simulink model "fuzzy_PD"  (R2022b)
settings: Solver=VariableStepAuto  StartTime=0.0  StopTime=400  RelTol=1e-3
libraries: fuzblock x1
settings Model: Creator=sophy  LastModifiedBy=sophy

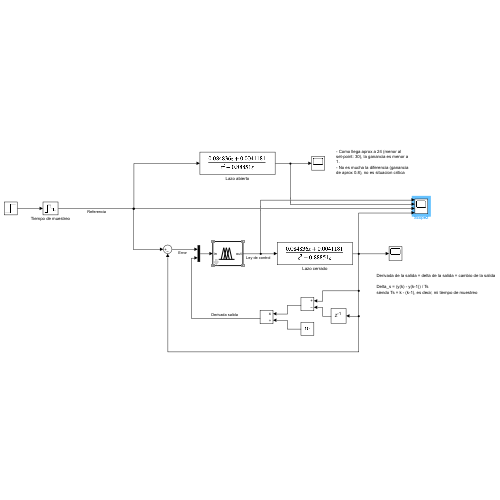
[thumbnail: Simulink's stored preview of the top-level diagram]
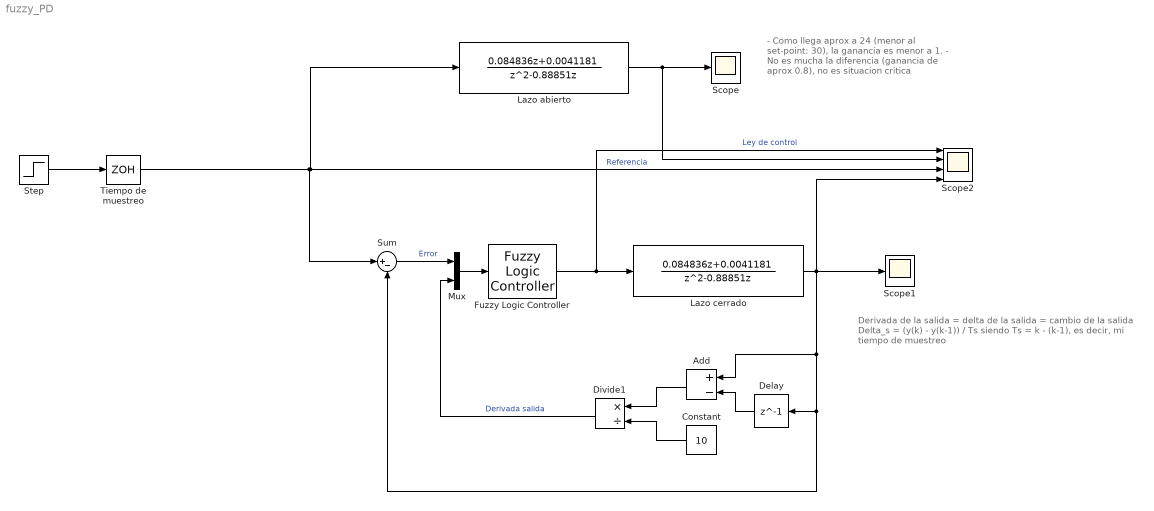
== system fuzzy_PD ==
  note: Derivada de la salida = delta de la salida = cambio de la salida
      |
      | Delta_s = (y(k) - y(k-1)) / Ts
      | siendo Ts = k - (k-1), es decir, mi tiempo de muestreo
  note: - Como llega aprox a 24 (menor al set-point: 30), la ganancia es menor a 1.
      | - No es mucha la diferencia (ganancia de aprox 0.8), no es situacion critica
  Add : Sum  Inputs=+-
  Constant : Constant  Value=10
  Delay : Delay  DelayLength=1
  Divide1 : Product  Inputs=*/
  Fuzzy Logic Controller : fuzblock/Fuzzy Logic  Controller  FIS=mamdanitype1  OutputSampleNumber=101  DataType=double  FuzzifiedInputs=off  RuleFiringStrengths=off  RuleOutputs=off  AggregatedOutputs=off  SimulateUsing=Interpreted execution  OutOfRangeInputValueMessage=warning  NoRuleFiredMessage=warning  EmptyOutputFuzzySetMessage=warning
  Lazo abierto : DiscreteTransferFcn  Numerator=[0.084836 0.0041181]  Denominator=[1 -0.88851 0]
  Lazo cerrado : DiscreteTransferFcn  Numerator=[0.084836 0.0041181]  Denominator=[1 -0.88851 0]
  Mux : Mux  Inputs=2
  Scope : Scope
  Scope1 : Scope
  Scope2 : Scope  NumInputPorts=4
  Step : Step  After=30  SampleTime=0
  Sum : Sum  Inputs=|+-
  Tiempo de muestreo : ZeroOrderHold  SampleTime=10
  wires:
  Step/1 -> Tiempo de muestreo/1
  Lazo abierto/1 -> Scope/1, Scope2/2
  Tiempo de muestreo/1 -> Sum/1, Scope2/3, Lazo abierto/1  "Referencia"
  Lazo cerrado/1 -> Scope2/4, Sum/2, Delay/1, Add/1, Scope1/1
  Fuzzy Logic Controller/1 -> Scope2/1, Lazo cerrado/1  "Ley de control"
  Sum/1 -> Mux/1  "Error"
  Mux/1 -> Fuzzy Logic Controller/1
  Add/1 -> Divide1/1
  Constant/1 -> Divide1/2
  Divide1/1 -> Mux/2  "Derivada salida"
  Delay/1 -> Add/2
